simulink model "Active_Suspension_2_Simulink"  (R2023b)
settings: Solver=VariableStepAuto  StartTime=0.0  StopTime=40.0  MaxStep=1e-4  RelTol=1e-3
values from neighbouring files (symbols this model uses):
  A = [0 1 0 0; -(kc_sse/mc_sse) -(cc_sse/mc_sse) (kc_sse/mc_sse) (cc_sse/mc_sse); 0 0 0 1; (kc_sse/mw_sse) (cc_sse/mw_sse) -((kc_sse + kw_sse)/mw_sse) -(cc_sse/mw_sse)]    [Active_Suspension_1.m]    (also in Active_Suspension_Control.m = [ 0 1 0 0; [-k_car -c_car k_car c_car]/m_car ; 0 0 0 1; [k_c; Active_With_Robust_Road.m; Extras.m; Robust_Active_Suspension_Control.m = [ 0 1 0 0; [-k_car -c_car k_car c_car]/m_car ; 0 0 0 1; [k_c)
  B = [0 0; (1/mc_sse) 0; 0 0; -(1/mw_sse) (kw_sse/ mw_sse)]    [Active_Suspension_1.m]    (also in Active_Suspension_Control.m = [ 0 0; 0 1/m_car ; 0 0 ; [-1 k_wheel]/m_wheel]; Active_With_Robust_Road.m; Extras.m; Robust_Active_Suspension_Control.m = [ 0 0; 0 1e3/m_car ; 0 0 ; [k_wheel -1e3]/m_wheel])
  C = [1 0 0 0]    [Active_Suspension_1.m]    (also in Active_Suspension_Control.m; Active_With_Robust_Road.m; Extras.m; Robust_Active_Suspension_Control.m = [1 0 0 0; 1 0 -1 0; A(2,:)])
  cc_1 = 30    [Extras.m]
  cc_2 = 30    [Extras.m]
  cw_2 = 10:10:70    [Extras.m]
  D = [0 0]    [Active_Suspension_1.m]    (also in Active_Suspension_Control.m; Active_With_Robust_Road.m; Extras.m; Robust_Active_Suspension_Control.m = [0 0; 0 0; B(2,:)])
  kc_1 = 23    [Extras.m]
  kc_2 = 23    [Extras.m]
  kw_1 = 700    [Extras.m]
  kw_2 = 700    [Extras.m]
  mc_1 = 60    [Extras.m]
  mc_2 = 60    [Extras.m]
  mw_1 = 12    [Extras.m]
  mw_2 = 12    [Extras.m]
  u1 = [uc; ud]    [Robust_With_Adaptive_Road.m]
settings Model: Creator=hkurt  LastModifiedBy=hkurt

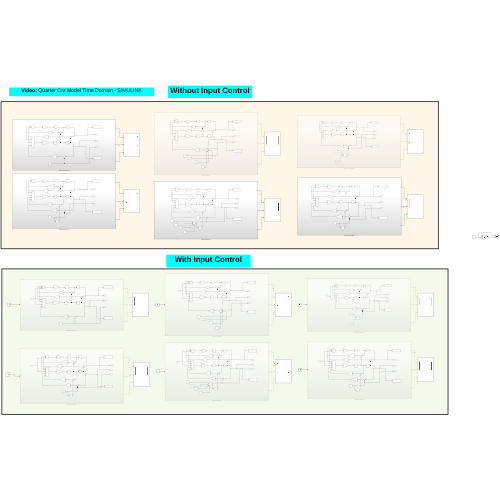
[thumbnail: Simulink's stored preview of the top-level diagram]
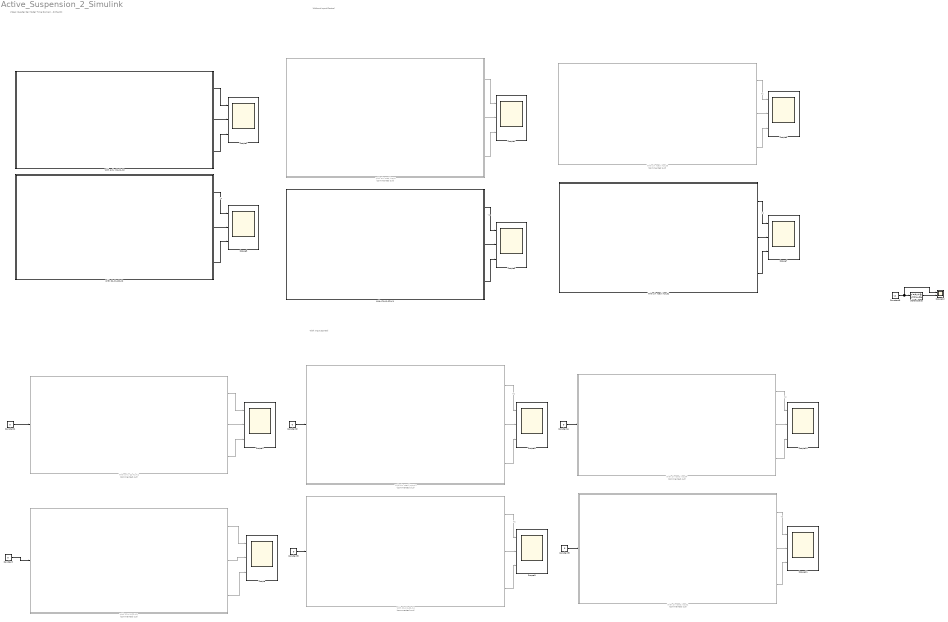
== system Active_Suspension_2_Simulink ==
  note: Yc
  note: Yc
  note: Yc
  note: Yc
  note: Yc
  note: Yc
  note: Yc
  note: Yc
  note: Without Input Control
  note: With Input Control
  note: Video: Quarter Car Model Time Domain - SIMULINK
  Constant{,1..5} (6 alike) : Constant  Value=0
  Constant6 : Constant  Value=u1
  Scope{,1..11} (12 alike) : Scope  NumInputPorts=3
  Scope12 : Scope  NumInputPorts=2
  State-Space : StateSpace  A=A  B=B  C=C  D=D  InitialCondition=0
  With C1-K1-C2-K1 : Subsystem
  With C1-K1-C2-K2 : Subsystem
  With C1-K1-C2-K3 : Subsystem  Commented=on
  With C1-K1-C2-K4 : Subsystem  Commented=on
  With only C1-K1-K1 : Subsystem  Commented=on
  With only C1-K1-K2 : Subsystem
  "With sin road input " : Subsystem  Commented=on
  With sin road input 1 : Subsystem  Commented=on
  With sin road input1 : Subsystem  Commented=on
  With sin road input2 : Subsystem
  With sin road input3 : Subsystem  Commented=on
  With sin road input4 : Subsystem  Commented=on
  wires:
  With C1-K1-C2-K3/1(Output) -> Scope/1  "Yc"
  With C1-K1-C2-K3/2(Output1) -> Scope/2  "Yw"
  With C1-K1-C2-K3/3(Output2) -> Scope/3  "X"
  Constant/1 -> With C1-K1-C2-K3/1(Input)
  Constant1/1 -> With only C1-K1-K1/1(Input)
  With only C1-K1-K1/1(Output) -> Scope1/1  "Yc"
  With only C1-K1-K1/2(Output1) -> Scope1/2  "Yw"
  With only C1-K1-K1/3(Output2) -> Scope1/3  "X"
  With only C1-K1-K2/1(Output) -> Scope2/1  "Yc"
  With only C1-K1-K2/2(Output1) -> Scope2/2  "Yw"
  With only C1-K1-K2/3(Output2) -> Scope2/3  "X"
  With C1-K1-C2-K2/1(Output) -> Scope3/1
  With C1-K1-C2-K2/2(Output1) -> Scope3/2  "Yw"
  With C1-K1-C2-K2/3(Output2) -> Scope3/3  "X"
  "With sin road input "/2(Output1) -> Scope4/2  "Yw"
  "With sin road input "/1(Output) -> Scope4/1  "Yc"
  "With sin road input "/3(Output2) -> Scope4/3  "X"
  With C1-K1-C2-K1/2(Output1) -> Scope5/2  "Yw"
  With C1-K1-C2-K1/1(Output) -> Scope5/1
  With C1-K1-C2-K1/3(Output2) -> Scope5/3  "X"
  With sin road input3/1(Output) -> Scope6/1
  With sin road input3/2(Output1) -> Scope6/2  "Yw"
  With sin road input3/3(Output2) -> Scope6/3  "X"
  With sin road input2/1(Output) -> Scope7/1
  With sin road input2/2(Output1) -> Scope7/2  "Yw"
  With sin road input2/3(Output2) -> Scope7/3  "X"
  With C1-K1-C2-K4/3(Output2) -> Scope9/3  "X"
  With sin road input 1/3(Output2) -> Scope8/3  "X"
  With sin road input 1/2(Output1) -> Scope8/2  "Yw"
  With sin road input 1/1(Output) -> Scope8/1
  With C1-K1-C2-K4/1(Output) -> Scope9/1
  With C1-K1-C2-K4/2(Output1) -> Scope9/2  "Yw"
  Constant2/1 -> With sin road input 1/1(Input)
  Constant3/1 -> With C1-K1-C2-K4/1(Input)
  With sin road input4/2(Output1) -> Scope10/2  "Yw"
  With sin road input4/3(Output2) -> Scope10/3  "X"
  With sin road input1/3(Output2) -> Scope11/3  "X"
  With sin road input1/1(Output) -> Scope11/1
  With sin road input1/2(Output1) -> Scope11/2  "Yw"
  With sin road input4/1(Output) -> Scope10/1
  Constant4/1 -> With sin road input4/1(Input)
  Constant5/1 -> With sin road input1/1(Input)
  State-Space/1 -> Scope12/2
  Constant6/1 -> Scope12/1, State-Space/1

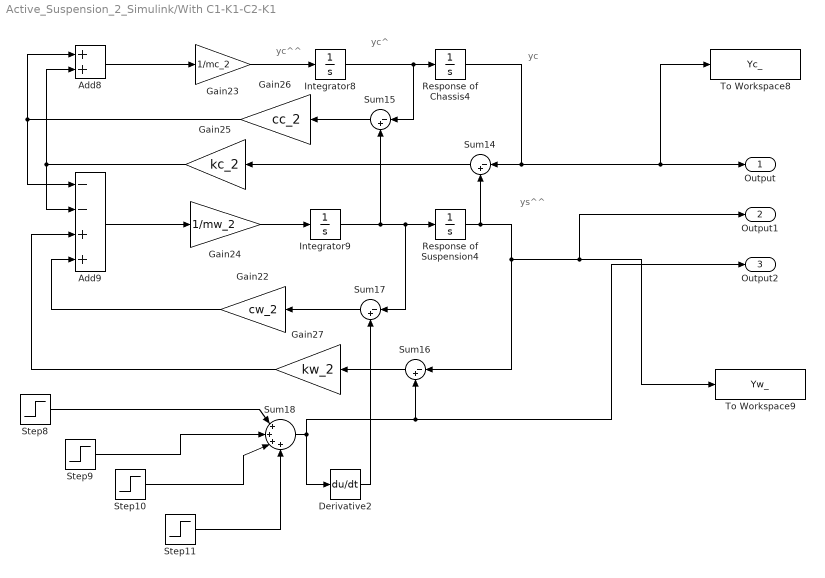
== system Active_Suspension_2_Simulink/With C1-K1-C2-K1 ==
  note: yc^^
  note: ys^^
  note: yc^
  note: yc
  Add8 : Sum
  Add9 : Sum  Inputs=--++
  Derivative2 : Derivative
  Gain22 : Gain  Gain=cw_2
  Gain23 : Gain  Gain=1/mc_2
  Gain24 : Gain  Gain=1/mw_2
  Gain25 : Gain  Gain=kc_2
  Gain26 : Gain  Gain=cc_2
  Gain27 : Gain  Gain=kw_2
  Integrator8 : Integrator
  Integrator9 : Integrator
  Response of Chassis4 : Integrator
  Response of Suspension4 : Integrator
  Step10 : Step  Time=15  After=-10  SampleTime=0
  Step11 : Step  Time=20  After=5  SampleTime=0
  Step8 : Step  Time=5  After=10  SampleTime=0
  Step9 : Step  Time=10  After=20  SampleTime=0
  Sum{14..17} (4 alike) : Sum  Inputs=|-+
  Sum18 : Sum  Inputs=|++++
  To Workspace8 : ToWorkspace  VariableName=Yc_  SaveFormat=Timeseries  SampleTime=-1
  To Workspace9 : ToWorkspace  VariableName=Yw_  SaveFormat=Timeseries  SampleTime=-1
  Output : Outport
  Output1 : Outport  Port=2
  Output2 : Outport  Port=3
  wires:
  Gain24/1 -> Integrator9/1
  Sum17/1 -> Gain22/1
  Step10/1 -> Sum18/3
  Gain22/1 -> Add9/4
  Sum16/1 -> Gain27/1
  Step9/1 -> Sum18/2
  Sum15/1 -> Gain26/1
  Step11/1 -> Sum18/4
  Integrator8/1 -> Sum15/1, Response of Chassis4/1
  Sum18/1 -> Output2/1, Sum16/2, Derivative2/1
  Integrator9/1 -> Sum15/2, Sum17/1, Response of Suspension4/1
  Gain25/1 -> Add9/2, Add8/2
  Derivative2/1 -> Sum17/2
  Sum14/1 -> Gain25/1
  Response of Chassis4/1 -> Sum14/1, Output/1, To Workspace8/1
  Add8/1 -> Gain23/1
  Step8/1 -> Sum18/1
  Response of Suspension4/1 -> Sum14/2, Sum16/1, Output1/1, To Workspace9/1
  Add9/1 -> Gain24/1
  Gain23/1 -> Integrator8/1
  Gain27/1 -> Add9/3
  Gain26/1 -> Add9/1, Add8/1

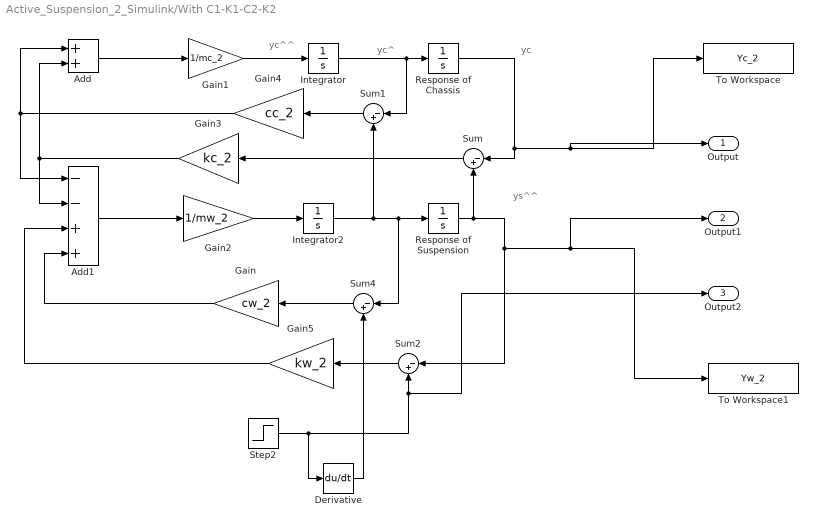
== system Active_Suspension_2_Simulink/With C1-K1-C2-K2 ==
  note: yc
  note: ys^^
  note: yc^
  note: yc^^
  Add : Sum
  Add1 : Sum  Inputs=--++
  Derivative : Derivative
  Gain : Gain  Gain=cw_2
  Gain1 : Gain  Gain=1/mc_2
  Gain2 : Gain  Gain=1/mw_2
  Gain3 : Gain  Gain=kc_2
  Gain4 : Gain  Gain=cc_2
  Gain5 : Gain  Gain=kw_2
  Integrator : Integrator
  Integrator2 : Integrator
  Response of Chassis : Integrator
  Response of Suspension : Integrator
  Step2 : Step  After=30  SampleTime=0
  Sum{,1..2,4} (4 alike) : Sum  Inputs=|-+
  To Workspace : ToWorkspace  VariableName=Yc_2  SaveFormat=Timeseries  SampleTime=-1
  To Workspace1 : ToWorkspace  VariableName=Yw_2  SaveFormat=Timeseries  SampleTime=-1
  Output : Outport
  Output1 : Outport  Port=2
  Output2 : Outport  Port=3
  wires:
  Add1/1 -> Gain2/1
  Gain1/1 -> Integrator/1
  Integrator/1 -> Sum1/1, Response of Chassis/1
  Gain3/1 -> Add1/2, Add/2
  Step2/1 -> Derivative/1, Sum2/2, Output2/1
  Sum1/1 -> Gain4/1
  Add/1 -> Gain1/1
  Gain4/1 -> Add1/1, Add/1
  Integrator2/1 -> Sum1/2, Sum4/1, Response of Suspension/1
  Gain2/1 -> Integrator2/1
  Response of Suspension/1 -> Sum/2, Sum2/1, Output1/1, To Workspace1/1
  Derivative/1 -> Sum4/2
  Gain5/1 -> Add1/3
  Sum4/1 -> Gain/1
  Sum/1 -> Gain3/1
  Gain/1 -> Add1/4
  Response of Chassis/1 -> Sum/1, Output/1, To Workspace/1
  Sum2/1 -> Gain5/1

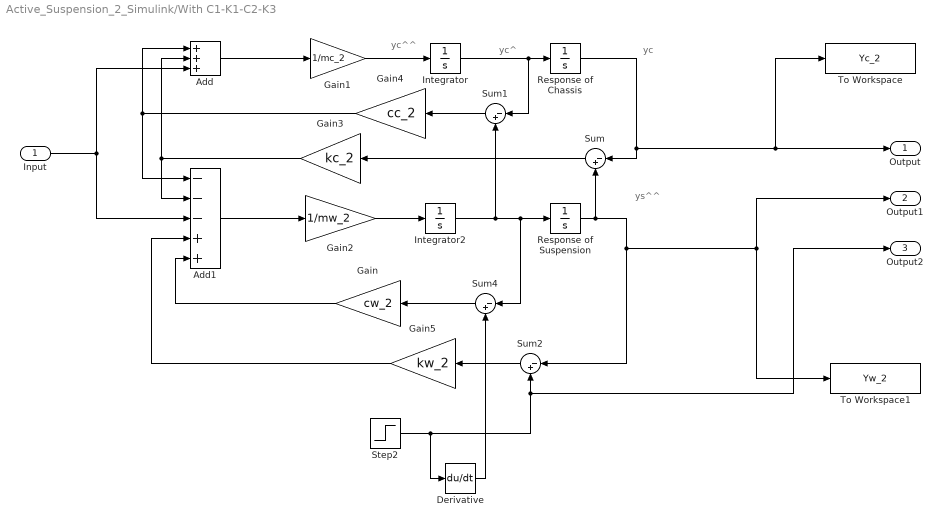
== system Active_Suspension_2_Simulink/With C1-K1-C2-K3 ==
  note: yc
  note: ys^^
  note: yc^
  note: yc^^
  Input : Inport
  Add : Sum  Inputs=+++
  Add1 : Sum  Inputs=---++
  Derivative : Derivative
  Gain : Gain  Gain=cw_2
  Gain1 : Gain  Gain=1/mc_2
  Gain2 : Gain  Gain=1/mw_2
  Gain3 : Gain  Gain=kc_2
  Gain4 : Gain  Gain=cc_2
  Gain5 : Gain  Gain=kw_2
  Integrator : Integrator
  Integrator2 : Integrator
  Response of Chassis : Integrator
  Response of Suspension : Integrator
  Step2 : Step  After=30  SampleTime=0
  Sum{,1..2,4} (4 alike) : Sum  Inputs=|-+
  To Workspace : ToWorkspace  VariableName=Yc_2  SaveFormat=Timeseries  SampleTime=-1
  To Workspace1 : ToWorkspace  VariableName=Yw_2  SaveFormat=Timeseries  SampleTime=-1
  Output : Outport
  Output1 : Outport  Port=2
  Output2 : Outport  Port=3
  wires:
  Add1/1 -> Gain2/1
  Gain1/1 -> Integrator/1
  Integrator/1 -> Sum1/1, Response of Chassis/1
  Gain3/1 -> Add1/2, Add/2
  Step2/1 -> Derivative/1, Output2/1, Sum2/2
  Sum1/1 -> Gain4/1
  Add/1 -> Gain1/1
  Gain4/1 -> Add1/1, Add/1
  Integrator2/1 -> Sum1/2, Sum4/1, Response of Suspension/1
  Gain2/1 -> Integrator2/1
  Response of Suspension/1 -> Sum/2, Sum2/1, Output1/1, To Workspace1/1
  Derivative/1 -> Sum4/2
  Gain5/1 -> Add1/4
  Sum4/1 -> Gain/1
  Sum/1 -> Gain3/1
  Gain/1 -> Add1/5
  Response of Chassis/1 -> Sum/1, To Workspace/1, Output/1
  Sum2/1 -> Gain5/1
  Input/1 -> Add1/3, Add/3

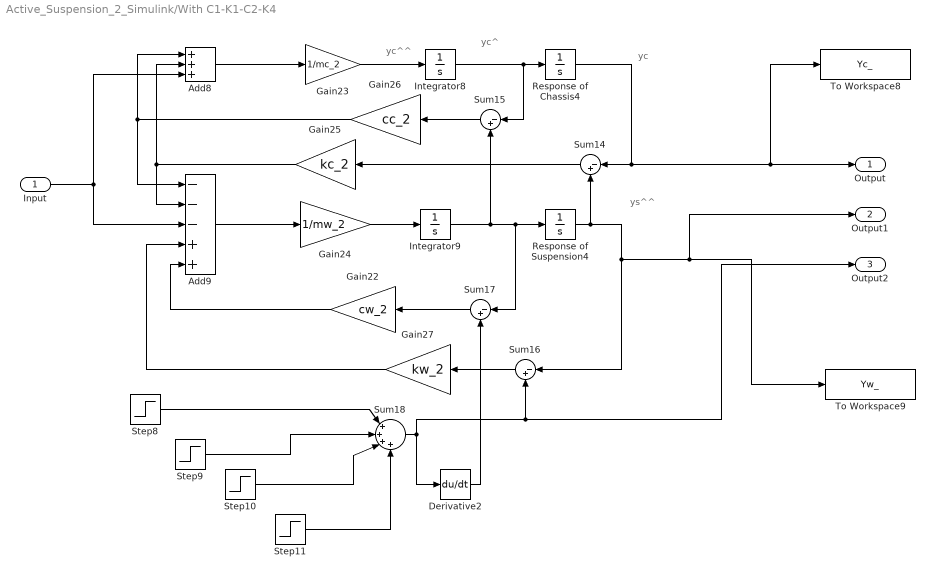
== system Active_Suspension_2_Simulink/With C1-K1-C2-K4 ==
  note: yc^^
  note: ys^^
  note: yc^
  note: yc
  Input : Inport
  Add8 : Sum  Inputs=+++
  Add9 : Sum  Inputs=---++
  Derivative2 : Derivative
  Gain22 : Gain  Gain=cw_2
  Gain23 : Gain  Gain=1/mc_2
  Gain24 : Gain  Gain=1/mw_2
  Gain25 : Gain  Gain=kc_2
  Gain26 : Gain  Gain=cc_2
  Gain27 : Gain  Gain=kw_2
  Integrator8 : Integrator
  Integrator9 : Integrator
  Response of Chassis4 : Integrator
  Response of Suspension4 : Integrator
  Step10 : Step  Time=15  After=-10  SampleTime=0
  Step11 : Step  Time=20  After=5  SampleTime=0
  Step8 : Step  Time=5  After=10  SampleTime=0
  Step9 : Step  Time=10  After=20  SampleTime=0
  Sum{14..17} (4 alike) : Sum  Inputs=|-+
  Sum18 : Sum  Inputs=|++++
  To Workspace8 : ToWorkspace  VariableName=Yc_  SaveFormat=Timeseries  SampleTime=-1
  To Workspace9 : ToWorkspace  VariableName=Yw_  SaveFormat=Timeseries  SampleTime=-1
  Output : Outport
  Output1 : Outport  Port=2
  Output2 : Outport  Port=3
  wires:
  Gain24/1 -> Integrator9/1
  Sum17/1 -> Gain22/1
  Step10/1 -> Sum18/3
  Gain22/1 -> Add9/5
  Sum16/1 -> Gain27/1
  Step9/1 -> Sum18/2
  Sum15/1 -> Gain26/1
  Step11/1 -> Sum18/4
  Integrator8/1 -> Sum15/1, Response of Chassis4/1
  Sum18/1 -> Output2/1, Sum16/2, Derivative2/1
  Integrator9/1 -> Sum15/2, Sum17/1, Response of Suspension4/1
  Gain25/1 -> Add9/2, Add8/2
  Derivative2/1 -> Sum17/2
  Sum14/1 -> Gain25/1
  Response of Chassis4/1 -> Sum14/1, Output/1, To Workspace8/1
  Add8/1 -> Gain23/1
  Step8/1 -> Sum18/1
  Response of Suspension4/1 -> Sum14/2, Sum16/1, Output1/1, To Workspace9/1
  Add9/1 -> Gain24/1
  Gain23/1 -> Integrator8/1
  Gain27/1 -> Add9/4
  Gain26/1 -> Add9/1, Add8/1
  Input/1 -> Add9/3, Add8/3

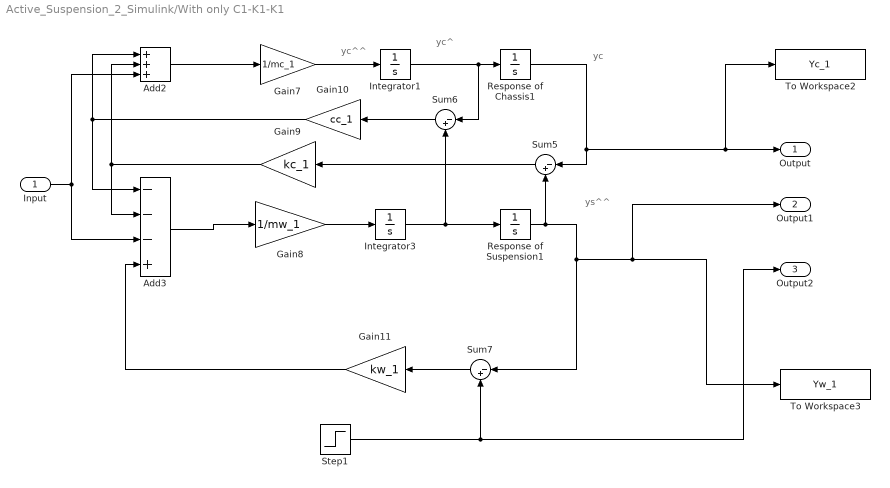
== system Active_Suspension_2_Simulink/With only C1-K1-K1 ==
  note: ys^^
  note: yc^^
  note: yc
  note: yc^
  Input : Inport
  Add2 : Sum  Inputs=+++
  Add3 : Sum  Inputs=---+
  Gain10 : Gain  Gain=cc_1
  Gain11 : Gain  Gain=kw_1
  Gain7 : Gain  Gain=1/mc_1
  Gain8 : Gain  Gain=1/mw_1
  Gain9 : Gain  Gain=kc_1
  Integrator1 : Integrator
  Integrator3 : Integrator
  Response of Chassis1 : Integrator
  Response of Suspension1 : Integrator
  Step1 : Step  After=30  SampleTime=0
  Sum5 : Sum  Inputs=|-+
  Sum6 : Sum  Inputs=|-+
  Sum7 : Sum  Inputs=|-+
  To Workspace2 : ToWorkspace  VariableName=Yc_1  SaveFormat=Timeseries  SampleTime=-1
  To Workspace3 : ToWorkspace  VariableName=Yw_1  SaveFormat=Timeseries  SampleTime=-1
  Output : Outport
  Output1 : Outport  Port=2
  Output2 : Outport  Port=3
  wires:
  Gain11/1 -> Add3/4
  Sum5/1 -> Gain9/1
  Add3/1 -> Gain8/1
  Response of Suspension1/1 -> Sum5/2, Sum7/1, Output1/1, To Workspace3/1
  Sum7/1 -> Gain11/1
  Integrator1/1 -> Sum6/1, Response of Chassis1/1
  Gain8/1 -> Integrator3/1
  Gain9/1 -> Add3/2, Add2/2
  Sum6/1 -> Gain10/1
  Response of Chassis1/1 -> Sum5/1, Output/1, To Workspace2/1
  Gain7/1 -> Integrator1/1
  Step1/1 -> Output2/1, Sum7/2
  Integrator3/1 -> Sum6/2, Response of Suspension1/1
  Add2/1 -> Gain7/1
  Gain10/1 -> Add3/1, Add2/1
  Input/1 -> Add2/3, Add3/3

== system Active_Suspension_2_Simulink/With only C1-K1-K2 ==
  note: ys^^
  note: yc^^
  note: yc
  note: yc^
  Add2 : Sum
  Add3 : Sum  Inputs=--+
  Gain10 : Gain  Gain=cc_1
  Gain11 : Gain  Gain=kw_1
  Gain7 : Gain  Gain=1/mc_1
  Gain8 : Gain  Gain=1/mw_1
  Gain9 : Gain  Gain=kc_1
  Integrator1 : Integrator
  Integrator3 : Integrator
  Response of Chassis1 : Integrator
  Response of Suspension1 : Integrator
  Step1 : Step  After=30  SampleTime=0
  Sum5 : Sum  Inputs=|-+
  Sum6 : Sum  Inputs=|-+
  Sum7 : Sum  Inputs=|-+
  To Workspace2 : ToWorkspace  VariableName=Yc_1  SaveFormat=Timeseries  SampleTime=-1
  To Workspace3 : ToWorkspace  VariableName=Yw_1  SaveFormat=Timeseries  SampleTime=-1
  Output : Outport
  Output1 : Outport  Port=2
  Output2 : Outport  Port=3
  wires:
  Gain11/1 -> Add3/3
  Sum5/1 -> Gain9/1
  Add3/1 -> Gain8/1
  Response of Suspension1/1 -> Sum5/2, Sum7/1, Output1/1, To Workspace3/1
  Sum7/1 -> Gain11/1
  Integrator1/1 -> Sum6/1, Response of Chassis1/1
  Gain8/1 -> Integrator3/1
  Gain9/1 -> Add3/2, Add2/2
  Sum6/1 -> Gain10/1
  Gain7/1 -> Integrator1/1
  Step1/1 -> Output2/1, Sum7/2
  Integrator3/1 -> Sum6/2, Response of Suspension1/1
  Add2/1 -> Gain7/1
  Gain10/1 -> Add3/1, Add2/1
  Response of Chassis1/1 -> Sum5/1, Output/1, To Workspace2/1

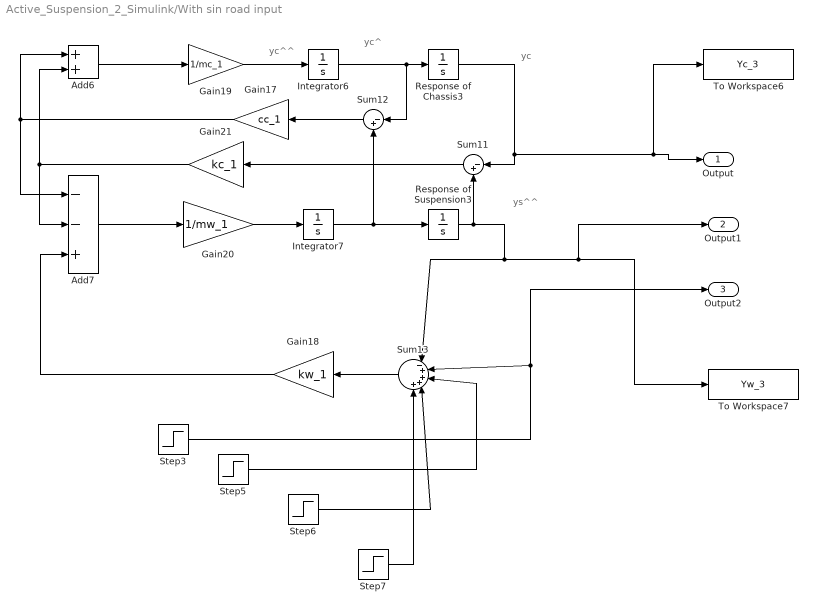
== system Active_Suspension_2_Simulink/With sin road input  ==
  note: yc^^
  note: yc^
  note: yc
  note: ys^^
  Add6 : Sum
  Add7 : Sum  Inputs=--+
  Gain17 : Gain  Gain=cc_1
  Gain18 : Gain  Gain=kw_1
  Gain19 : Gain  Gain=1/mc_1
  Gain20 : Gain  Gain=1/mw_1
  Gain21 : Gain  Gain=kc_1
  Integrator6 : Integrator
  Integrator7 : Integrator
  Response of Chassis3 : Integrator
  Response of Suspension3 : Integrator
  Step3 : Step  Time=5  After=10  SampleTime=0
  Step5 : Step  Time=10  After=20  SampleTime=0
  Step6 : Step  Time=15  After=-10  SampleTime=0
  Step7 : Step  Time=20  After=5  SampleTime=0
  Sum11 : Sum  Inputs=|-+
  Sum12 : Sum  Inputs=|-+
  Sum13 : Sum  Inputs=|-++++
  To Workspace6 : ToWorkspace  VariableName=Yc_3  SaveFormat=Timeseries  SampleTime=-1
  To Workspace7 : ToWorkspace  VariableName=Yw_3  SaveFormat=Timeseries  SampleTime=-1
  Output : Outport
  Output1 : Outport  Port=2
  Output2 : Outport  Port=3
  wires:
  Step7/1 -> Sum13/5
  Add6/1 -> Gain19/1
  Gain18/1 -> Add7/3
  Integrator6/1 -> Sum12/1, Response of Chassis3/1
  Sum12/1 -> Gain17/1
  Step3/1 -> Sum13/2, Output2/1
  Add7/1 -> Gain20/1
  Gain19/1 -> Integrator6/1
  Gain20/1 -> Integrator7/1
  Integrator7/1 -> Sum12/2, Response of Suspension3/1
  Response of Chassis3/1 -> Sum11/1, Output/1, To Workspace6/1
  Sum13/1 -> Gain18/1
  Response of Suspension3/1 -> Sum11/2, Sum13/1, Output1/1, To Workspace7/1
  Gain17/1 -> Add7/1, Add6/1
  Sum11/1 -> Gain21/1
  Step5/1 -> Sum13/3
  Step6/1 -> Sum13/4
  Gain21/1 -> Add7/2, Add6/2

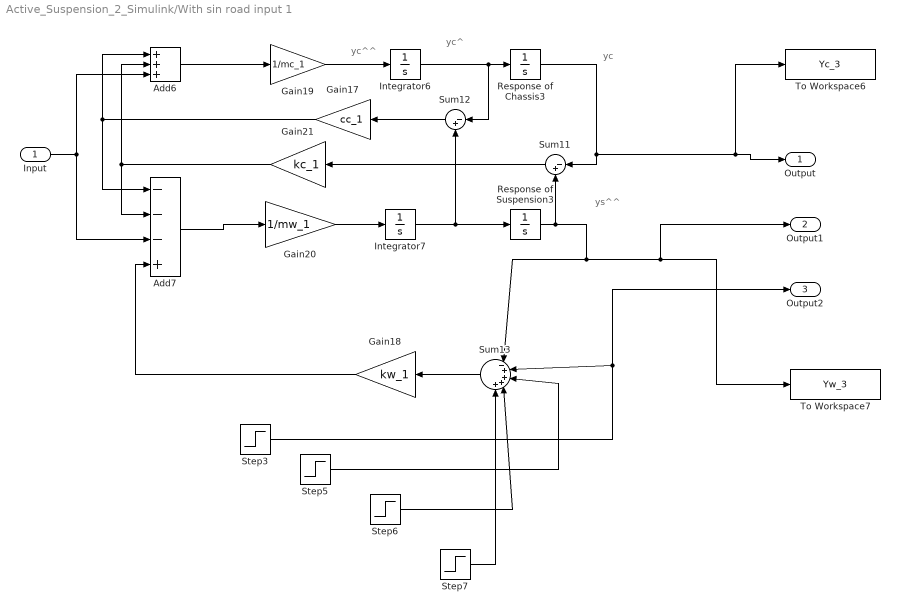
== system Active_Suspension_2_Simulink/With sin road input 1 ==
  note: yc^^
  note: yc^
  note: yc
  note: ys^^
  Input : Inport
  Add6 : Sum  Inputs=+++
  Add7 : Sum  Inputs=---+
  Gain17 : Gain  Gain=cc_1
  Gain18 : Gain  Gain=kw_1
  Gain19 : Gain  Gain=1/mc_1
  Gain20 : Gain  Gain=1/mw_1
  Gain21 : Gain  Gain=kc_1
  Integrator6 : Integrator
  Integrator7 : Integrator
  Response of Chassis3 : Integrator
  Response of Suspension3 : Integrator
  Step3 : Step  Time=5  After=10  SampleTime=0
  Step5 : Step  Time=10  After=20  SampleTime=0
  Step6 : Step  Time=15  After=-10  SampleTime=0
  Step7 : Step  Time=20  After=5  SampleTime=0
  Sum11 : Sum  Inputs=|-+
  Sum12 : Sum  Inputs=|-+
  Sum13 : Sum  Inputs=|-++++
  To Workspace6 : ToWorkspace  VariableName=Yc_3  SaveFormat=Timeseries  SampleTime=-1
  To Workspace7 : ToWorkspace  VariableName=Yw_3  SaveFormat=Timeseries  SampleTime=-1
  Output : Outport
  Output1 : Outport  Port=2
  Output2 : Outport  Port=3
  wires:
  Step7/1 -> Sum13/5
  Add6/1 -> Gain19/1
  Gain18/1 -> Add7/4
  Integrator6/1 -> Sum12/1, Response of Chassis3/1
  Sum12/1 -> Gain17/1
  Step3/1 -> Sum13/2, Output2/1
  Add7/1 -> Gain20/1
  Gain19/1 -> Integrator6/1
  Gain20/1 -> Integrator7/1
  Integrator7/1 -> Sum12/2, Response of Suspension3/1
  Response of Chassis3/1 -> Sum11/1, Output/1, To Workspace6/1
  Sum13/1 -> Gain18/1
  Response of Suspension3/1 -> Sum11/2, Sum13/1, Output1/1, To Workspace7/1
  Gain17/1 -> Add7/1, Add6/1
  Sum11/1 -> Gain21/1
  Step5/1 -> Sum13/3
  Step6/1 -> Sum13/4
  Gain21/1 -> Add7/2, Add6/2
  Input/1 -> Add7/3, Add6/3

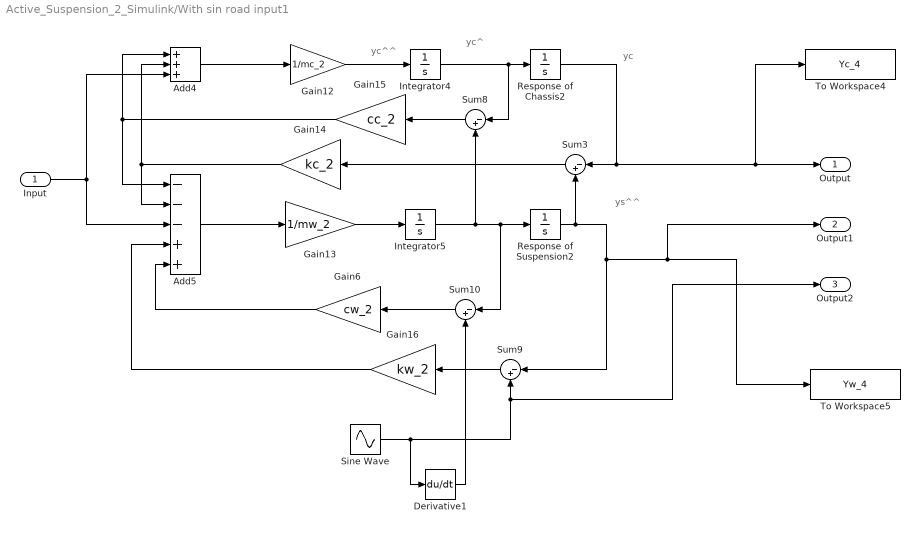
== system Active_Suspension_2_Simulink/With sin road input1 ==
  note: yc^^
  note: ys^^
  note: yc^
  note: yc
  Input : Inport
  Add4 : Sum  Inputs=+++
  Add5 : Sum  Inputs=---++
  Derivative1 : Derivative
  Gain12 : Gain  Gain=1/mc_2
  Gain13 : Gain  Gain=1/mw_2
  Gain14 : Gain  Gain=kc_2
  Gain15 : Gain  Gain=cc_2
  Gain16 : Gain  Gain=kw_2
  Gain6 : Gain  Gain=cw_2
  Integrator4 : Integrator
  Integrator5 : Integrator
  Response of Chassis2 : Integrator
  Response of Suspension2 : Integrator
  Sine Wave : Sin  Amplitude=30  Frequency=0.2  Phase=90*pi/360  SampleTime=0
  Sum{3,8..10} (4 alike) : Sum  Inputs=|-+
  To Workspace4 : ToWorkspace  VariableName=Yc_4  SaveFormat=Timeseries  SampleTime=-1
  To Workspace5 : ToWorkspace  VariableName=Yw_4  SaveFormat=Timeseries  SampleTime=-1
  Output : Outport
  Output1 : Outport  Port=2
  Output2 : Outport  Port=3
  wires:
  Response of Chassis2/1 -> Sum3/1, Output/1, To Workspace4/1
  Sum8/1 -> Gain15/1
  Gain15/1 -> Add5/1, Add4/1
  Gain6/1 -> Add5/5
  Gain13/1 -> Integrator5/1
  Sum9/1 -> Gain16/1
  Gain14/1 -> Add5/2, Add4/2
  Sum10/1 -> Gain6/1
  Sine Wave/1 -> Derivative1/1, Sum9/2, Output2/1
  Derivative1/1 -> Sum10/2
  Integrator5/1 -> Sum8/2, Sum10/1, Response of Suspension2/1
  Gain16/1 -> Add5/4
  Sum3/1 -> Gain14/1
  Add4/1 -> Gain12/1
  Integrator4/1 -> Sum8/1, Response of Chassis2/1
  Add5/1 -> Gain13/1
  Response of Suspension2/1 -> Sum3/2, Sum9/1, Output1/1, To Workspace5/1
  Gain12/1 -> Integrator4/1
  Input/1 -> Add5/3, Add4/3

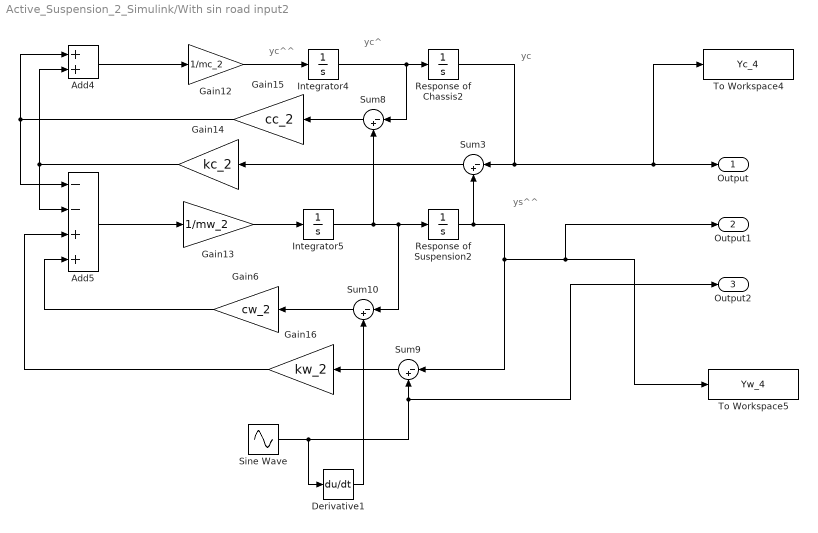
== system Active_Suspension_2_Simulink/With sin road input2 ==
  note: yc^^
  note: ys^^
  note: yc^
  note: yc
  Add4 : Sum
  Add5 : Sum  Inputs=--++
  Derivative1 : Derivative
  Gain12 : Gain  Gain=1/mc_2
  Gain13 : Gain  Gain=1/mw_2
  Gain14 : Gain  Gain=kc_2
  Gain15 : Gain  Gain=cc_2
  Gain16 : Gain  Gain=kw_2
  Gain6 : Gain  Gain=cw_2
  Integrator4 : Integrator
  Integrator5 : Integrator
  Response of Chassis2 : Integrator
  Response of Suspension2 : Integrator
  Sine Wave : Sin  Amplitude=30  Frequency=0.2  Phase=90*pi/360  SampleTime=0
  Sum{3,8..10} (4 alike) : Sum  Inputs=|-+
  To Workspace4 : ToWorkspace  VariableName=Yc_4  SaveFormat=Timeseries  SampleTime=-1
  To Workspace5 : ToWorkspace  VariableName=Yw_4  SaveFormat=Timeseries  SampleTime=-1
  Output : Outport
  Output1 : Outport  Port=2
  Output2 : Outport  Port=3
  wires:
  Response of Chassis2/1 -> Sum3/1, Output/1, To Workspace4/1
  Sum8/1 -> Gain15/1
  Gain15/1 -> Add5/1, Add4/1
  Gain6/1 -> Add5/4
  Gain13/1 -> Integrator5/1
  Sum9/1 -> Gain16/1
  Gain14/1 -> Add5/2, Add4/2
  Sum10/1 -> Gain6/1
  Sine Wave/1 -> Derivative1/1, Sum9/2, Output2/1
  Derivative1/1 -> Sum10/2
  Integrator5/1 -> Sum8/2, Sum10/1, Response of Suspension2/1
  Gain16/1 -> Add5/3
  Sum3/1 -> Gain14/1
  Add4/1 -> Gain12/1
  Integrator4/1 -> Sum8/1, Response of Chassis2/1
  Add5/1 -> Gain13/1
  Response of Suspension2/1 -> Sum3/2, Sum9/1, Output1/1, To Workspace5/1
  Gain12/1 -> Integrator4/1

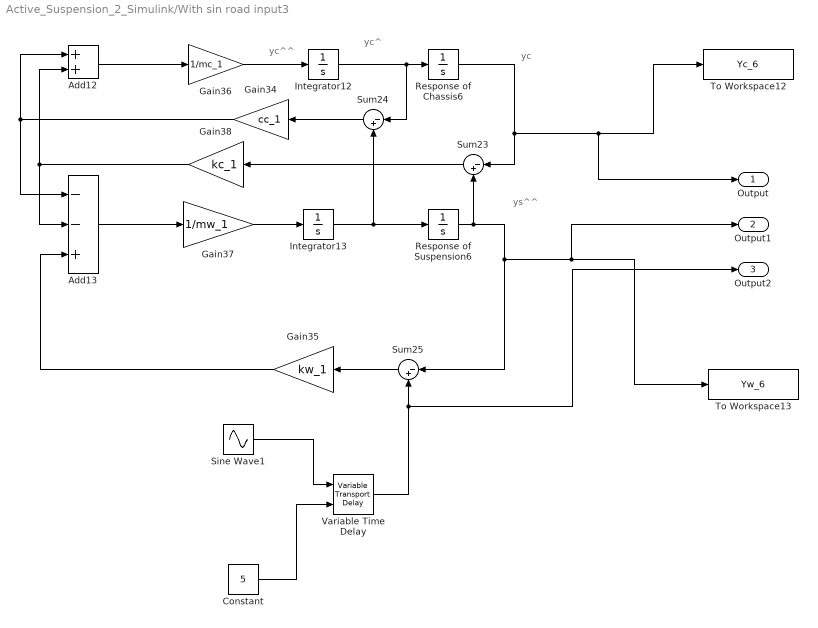
== system Active_Suspension_2_Simulink/With sin road input3 ==
  note: yc^^
  note: yc^
  note: yc
  note: ys^^
  Add12 : Sum
  Add13 : Sum  Inputs=--+
  Constant : Constant  Value=5
  Gain34 : Gain  Gain=cc_1
  Gain35 : Gain  Gain=kw_1
  Gain36 : Gain  Gain=1/mc_1
  Gain37 : Gain  Gain=1/mw_1
  Gain38 : Gain  Gain=kc_1
  Integrator12 : Integrator
  Integrator13 : Integrator
  Response of Chassis6 : Integrator
  Response of Suspension6 : Integrator
  Sine Wave1 : Sin  Amplitude=30  Frequency=0.2  SampleTime=0
  Sum23 : Sum  Inputs=|-+
  Sum24 : Sum  Inputs=|-+
  Sum25 : Sum  Inputs=|-+
  To Workspace12 : ToWorkspace  VariableName=Yc_6  SaveFormat=Timeseries  SampleTime=-1
  To Workspace13 : ToWorkspace  VariableName=Yw_6  SaveFormat=Timeseries  SampleTime=-1
  Variable Time Delay : VariableTransportDelay  MaximumDelay=10
  Output : Outport
  Output1 : Outport  Port=2
  Output2 : Outport  Port=3
  wires:
  Sum25/1 -> Gain35/1
  Integrator12/1 -> Sum24/1, Response of Chassis6/1
  Sum24/1 -> Gain34/1
  Response of Suspension6/1 -> Sum23/2, Sum25/1, Output1/1, To Workspace13/1
  Response of Chassis6/1 -> Output/1, To Workspace12/1, Sum23/1
  Sum23/1 -> Gain38/1
  Integrator13/1 -> Sum24/2, Response of Suspension6/1
  Gain37/1 -> Integrator13/1
  Add13/1 -> Gain37/1
  Gain35/1 -> Add13/3
  Gain34/1 -> Add13/1, Add12/1
  Gain36/1 -> Integrator12/1
  Sine Wave1/1 -> Variable Time Delay/1
  Gain38/1 -> Add13/2, Add12/2
  Add12/1 -> Gain36/1
  Constant/1 -> Variable Time Delay/2
  Variable Time Delay/1 -> Output2/1, Sum25/2

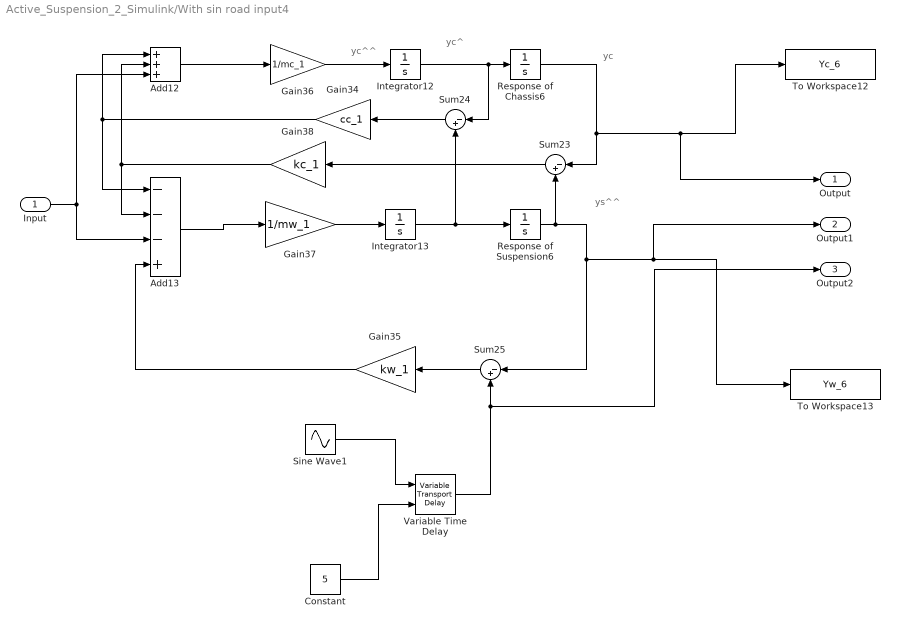
== system Active_Suspension_2_Simulink/With sin road input4 ==
  note: yc^^
  note: yc^
  note: yc
  note: ys^^
  Input : Inport
  Add12 : Sum  Inputs=+++
  Add13 : Sum  Inputs=---+
  Constant : Constant  Value=5
  Gain34 : Gain  Gain=cc_1
  Gain35 : Gain  Gain=kw_1
  Gain36 : Gain  Gain=1/mc_1
  Gain37 : Gain  Gain=1/mw_1
  Gain38 : Gain  Gain=kc_1
  Integrator12 : Integrator
  Integrator13 : Integrator
  Response of Chassis6 : Integrator
  Response of Suspension6 : Integrator
  Sine Wave1 : Sin  Amplitude=30  Frequency=0.2  SampleTime=0
  Sum23 : Sum  Inputs=|-+
  Sum24 : Sum  Inputs=|-+
  Sum25 : Sum  Inputs=|-+
  To Workspace12 : ToWorkspace  VariableName=Yc_6  SaveFormat=Timeseries  SampleTime=-1
  To Workspace13 : ToWorkspace  VariableName=Yw_6  SaveFormat=Timeseries  SampleTime=-1
  Variable Time Delay : VariableTransportDelay  MaximumDelay=10
  Output : Outport
  Output1 : Outport  Port=2
  Output2 : Outport  Port=3
  wires:
  Sum25/1 -> Gain35/1
  Integrator12/1 -> Sum24/1, Response of Chassis6/1
  Sum24/1 -> Gain34/1
  Response of Suspension6/1 -> Sum23/2, Sum25/1, Output1/1, To Workspace13/1
  Response of Chassis6/1 -> Output/1, To Workspace12/1, Sum23/1
  Sum23/1 -> Gain38/1
  Integrator13/1 -> Sum24/2, Response of Suspension6/1
  Gain37/1 -> Integrator13/1
  Add13/1 -> Gain37/1
  Gain35/1 -> Add13/4
  Gain34/1 -> Add13/1, Add12/1
  Gain36/1 -> Integrator12/1
  Sine Wave1/1 -> Variable Time Delay/1
  Gain38/1 -> Add13/2, Add12/2
  Add12/1 -> Gain36/1
  Constant/1 -> Variable Time Delay/2
  Variable Time Delay/1 -> Output2/1, Sum25/2
  Input/1 -> Add13/3, Add12/3
